simulink model "Q10"  (R2018a)
settings: Solver=VariableStepAuto  StartTime=0.0  StopTime=100  RelTol=1e-3
values from neighbouring files (symbols this model uses):
  A = [0.110571547291 0.471247754055 0.0249955131485 2.58943408161e-06 -0.326108592505 0.861622655316 0.0987425683373 1.02293307698e-05 -0.0747829687831 -0.0317325850518 0.998316867847 0.000207017546418 ... (16 elements, 4x4)]    [Q6.mat]    (also in SteelMillControl10.m = DiscPlant.A; SteelMillControl11.m = DiscPlant.A; SteelMillControl12.m = DiscPlant.A; SteelMillControl12lqr.m = DiscPlant.A)
  B = [0.00184081153928 0.000781109785891 4.14309453057e-05 4.29207838905e-09]    [Q6.mat]    (also in SteelMillControl10.m = DiscPlant.B; SteelMillControl11.m = DiscPlant.B; SteelMillControl12.m = DiscPlant.B; SteelMillControl12lqr.m = DiscPlant.B)
  C = [6.47358520402e-07 2.55733269246e-06 5.17543866044e-05 0.5]    [Q6.mat]    (also in SteelMillControl10.m = DiscPlant.C; SteelMillControl11.m = DiscPlant.C; SteelMillControl12.m = DiscPlant.C; SteelMillControl12lqr.m = DiscPlant.C)
  h = 9    [OlaSoup.m]    (also in Q3.mat = 0.0153022172533; Q6.mat = 0.03257469729; Q9disc.mat = 0.532796640949; SteelMillControl11.m = stepRes.RiseTime/11)
  K = [378.478532375 741.649236937 3450.29104505 3374760.11938]    [Q6.mat]    (also in SteelMillControl10.m = place(A,B,dp); SteelMillControl12.m = place(A,B,dp); SteelMillControl5.m = place(A,B,dp); SteelMillControl6.m = place(A,B,dp))
  Lcorr = inv(dcgain(ss(A-B*K,B,C,D,h)))    [SteelMillControl10.m]    (also in SteelMillControl11.m; SteelMillControl12.m; SteelMillControl12lqr.m; SteelMillControl5.m)
  xinit = [-17 5 -8 0.5]    [Q6.mat]    (also in SteelMillControl10.m = [0 0 0 0]; SteelMillControl11.m = [0 0 0 0]; SteelMillControl12.m = [0 0 0 0]; SteelMillControl12lqr.m = [0 0 0 0])
settings Model: Creator=bakos  LastModifiedBy=bakos
settings SolverCC: DecoupledContinuousIntegration=on  MinimalZcImpactIntegration=on

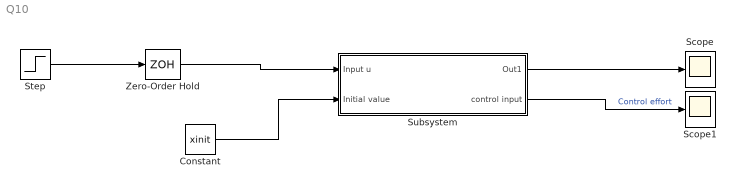
== system Q10 ==
  Constant : Constant  Value=xinit
  Scope : Scope
  Scope1 : Scope
  Step : Step  Time=0  SampleTime=0
  Subsystem : Subsystem
  Zero-Order Hold : ZeroOrderHold  SampleTime=h
  wires:
  Step/1 -> Zero-Order Hold/1
  Subsystem/1(Out1) -> Scope/1
  Subsystem/2(control input) -> Scope1/1  "Control effort"
  Constant/1 -> Subsystem/2(Initial value)
  Zero-Order Hold/1 -> Subsystem/1(Input u)

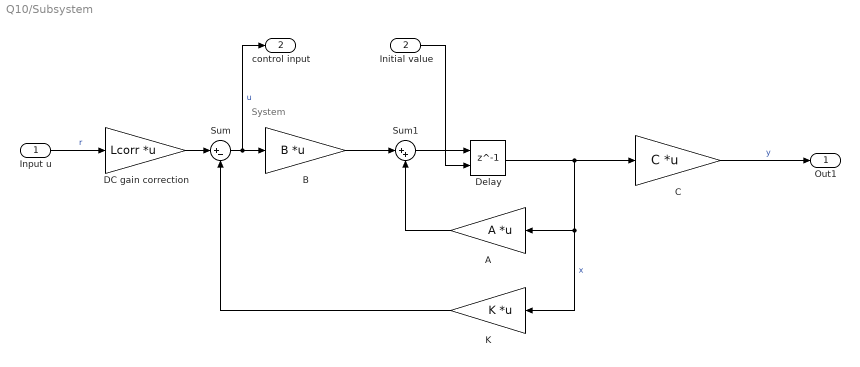
== system Q10/Subsystem ==
  note: System
  Input u : Inport
  Initial value : Inport  Port=2
  A : Gain  Gain=A  Multiplication=Matrix(K*u)
  B : Gain  Gain=B  Multiplication=Matrix(K*u)
  C : Gain  Gain=C  Multiplication=Matrix(K*u)
  DC gain correction : Gain  Gain=Lcorr  Multiplication=Matrix(K*u)
  Delay : Delay  DelayLength=1  InitialConditionSource=Input port  InitialCondition=0  SampleTime=h
      settings: InputPortMap=u0,p4
  K : Gain  Gain=K  Multiplication=Matrix(K*u)
  Sum : Sum  Inputs=|+-
  Sum1 : Sum  Inputs=|++
  Out1 : Outport
  control input : Outport  Port=2
  wires:
  Sum/1 -> control input/1, B/1  "u"
  B/1 -> Sum1/1
  Sum1/1 -> Delay/1
  Delay/1 -> A/1, K/1, C/1  "x"
  A/1 -> Sum1/2
  DC gain correction/1 -> Sum/1
  Input u/1 -> DC gain correction/1  "r"
  Initial value/1 -> Delay/2
  K/1 -> Sum/2
  C/1 -> Out1/1  "y"
